simulink model "Anfis_base_robot"  (R2019a)
settings: Solver=FixedStepAuto  StartTime=0.0  StopTime=inf  FixedStep=sampleTime  RelTol=1e-3
PreLoadFcn:
  | % Simulation parameters
  | load exampleMap
  | sampleTime = 0.05;
  | 
  | % Robot parameters
  | wheelRadius = 0.025;
  | robotRadius = 0.35;
  | 
  | % Lidar parameters
  | sensorOffset = [0,0];
  | scanAngles = linspace(-pi/2,pi/2,9)';
  | maxRange = 5;
libraries: neural x55, mobileRoboticsLib x10, fuzblock x1
(part 2 of 2)

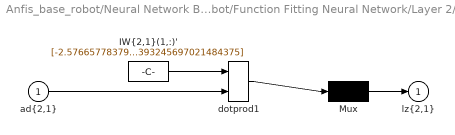
== system Anfis_base_robot/Neural Network Base RObot/Function Fitting Neural Network/Layer 2/LW{2,1} ==
  "ad{2,1}" : Inport  PortDimensions=50
      mask Display: e = 0.06;c1 = [120 230 180]/255;c2 = ([120 230 180]+0)/(256+128);c3 = ([120 230 180]+128)/(256+128);patch([0 1 1 0],[0 0 1 1],c1);patch([0 1 1 1-e 1-e 0+e],[0 0 1 1-e 0+e 0+e],c2);patch([0 0 1 1-e 0+e 0+e],[0 1 1 1-e 1-e 0+e],c3);plot([0 1 1 0 0],[0 0 1 1 0]);
  "IW{2,1}(1,:)'" : Constant  Value=[-2.57665778379313525903171466779895126819610595703125;0.2162823589462231910207634655307629145681858062744140625;-1.7656336646078598651143920506001450121402740478515625;1.9835078542767003995095365098677575588226318359375;-2.86175660155843214482729308656416833400726318359375;1.2225287887795002195190363636356778442859649658203125;-0.01017179809166622421467973680364593747071921825408935546875;0.8174787260377958109103246897575445473194122314453125;-0.6575146938363334303545570946880616247653961181640625;1.368671823745845284037159217405132949352264404296875;1.88504510307783146316751299309544265270233154296875;-2.09974673000754474827544981963001191616058349609375;0.613453109095142057327620932483114302158355712890625;0.50397133812463856816776797131751663982868194580078125;-3.01461324571703048746940112323500216007232666015625;3.208154391184654397051190244383178651332855224609375;-0.046896192246814467907700674231818993575870990753173828125;0.027235593019131969227952794199154595844447612762451171875;7.51224346836344469835466952645219862461090087890625;0.1313029942324970278377804788760840892791748046875;4.54839212946786464186743614845909178256988525390625;-2.52307630627870604911322516272775828838348388671875;-0.207491524320921438828690952504985034465789794921875;3.31862786312534563393228381755761802196502685546875;4.45817431056569812852785616996698081493377685546875;9.2950872179558956531764124520123004913330078125;-8.7238904538614843175992064061574637889862060546875;4.438766300466188141626844299025833606719970703125;-3.634026749860586047446986412978731095790863037109375;9.196892247438594125696909031830728054046630859375;9.1311201056973327894183967146091163158416748046875;0.1301483598886149783968591009397641755640506744384765625;-5.30938458527440371170769140007905662059783935546875;5.79635277529703074606004520319402217864990234375;-6.61622124977919501276346636586822569370269775390625;1.8919769309334952822609920985996723175048828125;0.344401068411469057917173586247372440993785858154296875;2.545753612416472577706372248940169811248779296875;0.604157513748693641986164948320947587490081787109375;0.50568046966589552670967577796545810997486114501953125;1.4744426041267593152639392428682185709476470947265625;-1.6068726171980223238477947234059683978557586669921875;-0.38759776960422775982095799918170087039470672607421875;0.365201367386207176313206446138792671263217926025390625;9.1826252838374440301549839205108582973480224609375;-0.0640566258095009999351532314904034137725830078125;-3.36696952956500439313458628021180629730224609375;-8.775751024024753377261731657199561595916748046875;-8.416398040424464710440588532947003841400146484375;9.8229817865662507614388232468627393245697021484375]
      mask Display: e = 0.06;c1 = [120 150 230]/255;c2 = ([120 150 230]+0)/383;c3 = ([120 150 230]+128)/383;patch([0 1 1 0],[0 0 1 1],c1);patch([0 1 1 1-e 1-e 0+e],[0 0 1 1-e 0+e 0+e],c2);patch([0 0 1 1-e 0+e 0+e],[0 1 1 1-e 1-e 0+e],c3);plot([0 1 1 0 0],[0 0 1 1 0]);disp('weights');
  Mux : Mux  Inputs=1
      mask Display: e = 0.06;c1 = [120 150 230]/255;c2 = ([120 150 230]+0)/383;c3 = ([120 150 230]+128)/383;patch([0 1 1 0],[0 0 1 1],c1);patch([0 1 1 1-e 1-e 0+e],[0 0 1 1-e 0+e 0+e],c2);patch([0 0 1 1-e 0+e 0+e],[0 1 1 1-e 1-e 0+e],c3);plot([0 1 1 0 0],[0 0 1 1 0]);disp('Mux');
  dotprod1 : neural/Weight Functions/dotprod
      settings: SourceProductName=MATLAB Runtime - Deep Learning Toolbox  SourceProductBaseCode=Missing
  "lz{2,1}" : Outport
      mask Display: e = 0.06;c1 = [120 230 180]/255;c2 = ([120 230 180]+0)/(256+128);c3 = ([120 230 180]+128)/(256+128);patch([0 1 1 0],[0 0 1 1],c1);patch([0 1 1 1-e 1-e 0+e],[0 0 1 1-e 0+e 0+e],c2);patch([0 0 1 1-e 0+e 0+e],[0 1 1 1-e 1-e 0+e],c3);plot([0 1 1 0 0],[0 0 1 1 0]);
  wires:
  "IW{2,1}(1,:)'"/1 -> dotprod1/1
  "ad{2,1}"/1 -> dotprod1/2
  dotprod1/1 -> Mux/1
  Mux/1 -> "lz{2,1}"/1

== stateflow chart Anfis_base_robot/Neural Network Base RObot/Obstacle Avoidance Logic2 ==
  state MainState [parallel]
    en,du:
    validIdx = ~isnan(ranges);
    validRanges = ranges(validIdx);
    validAngles = angles(validIdx);
    avgAngle = mean(validAngles./validRanges);
    settings: executionOrder=1
  data: angles input; ranges input; validIdx local; validAngles local size=numel(scanAngles); validRanges output size=numel(scanAngles); avgAngle output

== stateflow chart Anfis_base_robot/Hardcoded /Obstacle Avoidance Logic2 ==
  state MainState [parallel]
    en,du:
    validIdx = ~isnan(ranges);
    validRanges = ranges(validIdx);
    validAngles = angles(validIdx);
    settings: executionOrder=1
    state Turn
      en,du:
      avgAngle = mean(validAngles./validRanges);
      state Left
        en, du:
        w = [0;12.5];
      state Right
        en, du:
        w = [12.5;0];
      (default) -> (junction 39)
      (junction 39) -> Left [order 1] : [avgAngle < 0]
      (junction 39) -> (junction 43) [order 2]
      Left -> Right : [after(1,sec) && ...
          | avgAngle > 0]
      Right -> Left : [after(1,sec) && ...
          | avgAngle < 0]
      (junction 43) -> Right
    state GoStraight
      en:
      w = [25; 25];
    (default) -> GoStraight
    GoStraight -> Turn : [any(validRanges<=1)]
    Turn -> GoStraight : [all(validRanges>1)]
  data: angles input; w output; ranges input; validRanges local size=numel(scanAngles); validIdx local; validAngles local size=numel(scanAngles); avgAngle local

== matlab function Anfis_base_robot/Neural Network Base RObot/Direction to speed conversion ==
  data: u input; y output
function y = fcn(u)
if (u>0.3)
    y=[30,0];
elseif(u<-0.3)
    y=[0,30];
else
    y=[30,30];
end

== matlab function Anfis_base_robot/AnFIS Base Robot/MATLAB Function ==
  data: left input; Direction output; right input
function Direction = fcn(left, right)
if (left==right)
    Direction=0;
elseif (left>right)
    Direction=1;
else
    Direction=-1;
end

== matlab function Anfis_base_robot/AnFIS Base Robot/Direction to speed conversion ==
  data: u input; y output
function y = fcn(u)
if (u>0.3)
    y=[30,0];
elseif(u<-0.3)
    y=[0,30];
else
    y=[30,30];
end

== matlab function Anfis_base_robot/Neural Network Base RObot/MATLAB Function ==
  data: left input; Direction output; right input
function Direction = fcn(left, right)
if (left==right)
    Direction=0;
elseif (left>right)
    Direction=1;
else
    Direction=-1;
end

== stateflow chart Anfis_base_robot/AnFIS Base Robot/Obstacle Avoidance Logic2 ==
  state MainState [parallel]
    en,du:
    validIdx = ~isnan(ranges);
    validRanges = ranges(validIdx);
    validAngles = angles(validIdx);
    avgAngle = mean(validAngles./validRanges);
    settings: executionOrder=1
  data: angles input; ranges input; validIdx local; validAngles local size=numel(scanAngles); validRanges output size=numel(scanAngles); avgAngle output
